simulink model "underactuated_model"  (R2023b)
settings: Solver=VariableStepAuto  StartTime=0.0  StopTime=10.0  RelTol=1e-6
values from neighbouring files (symbols this model uses):
  h0 = 0.3    [how_do_limits_affect_convergence.m]    (also in run_underactuated_model.m)
settings Model: Creator=Aaron  LastModifiedBy=Aaron

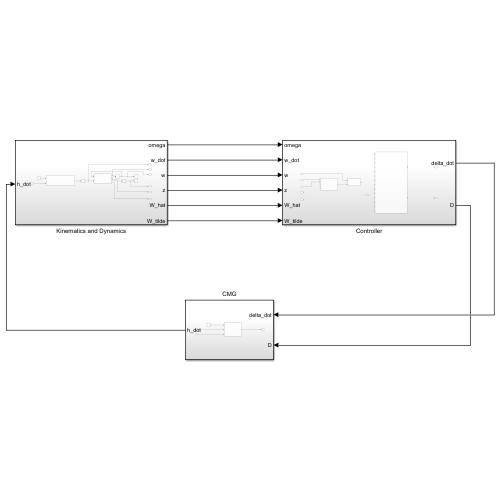
[thumbnail: Simulink's stored preview of the top-level diagram]
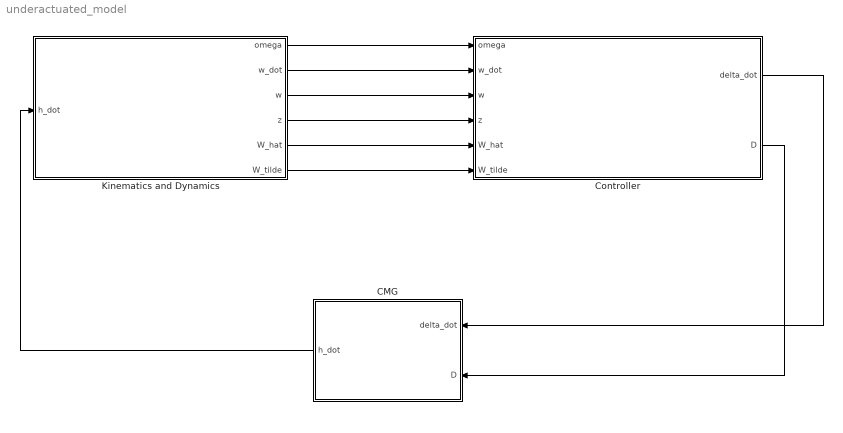
== system underactuated_model ==
  CMG : Subsystem
  Controller : Subsystem
  Kinematics and Dynamics : Subsystem
  wires:
  Kinematics and Dynamics/1(omega) -> Controller/1(omega)
  Kinematics and Dynamics/3(w) -> Controller/3(w)
  Kinematics and Dynamics/4(z) -> Controller/4(z)
  Kinematics and Dynamics/2(w_dot) -> Controller/2(w_dot)
  Kinematics and Dynamics/5(W_hat) -> Controller/5(W_hat)
  Kinematics and Dynamics/6(W_tilde) -> Controller/6(W_tilde)
  Controller/1(delta_dot) -> CMG/1(delta_dot)
  Controller/2(D) -> CMG/2(D)
  CMG/1(h_dot) -> Kinematics and Dynamics/1(h_dot)

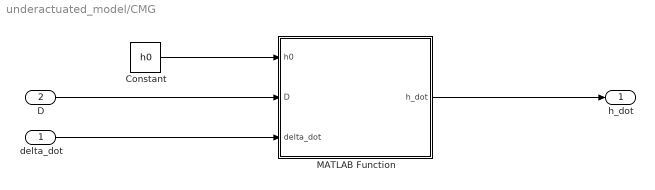
== system underactuated_model/CMG ==
  delta_dot : Inport
  D : Inport  Port=2
  Constant : Constant  Value=h0
  MATLAB Function : MATLAB Function  TreatAsAtomicUnit=on
  h_dot : Outport
  wires:
  delta_dot/1 -> MATLAB Function/3(delta_dot)
  D/1 -> MATLAB Function/2(D)
  MATLAB Function/1(h_dot) -> h_dot/1
  Constant/1 -> MATLAB Function/1(h0)

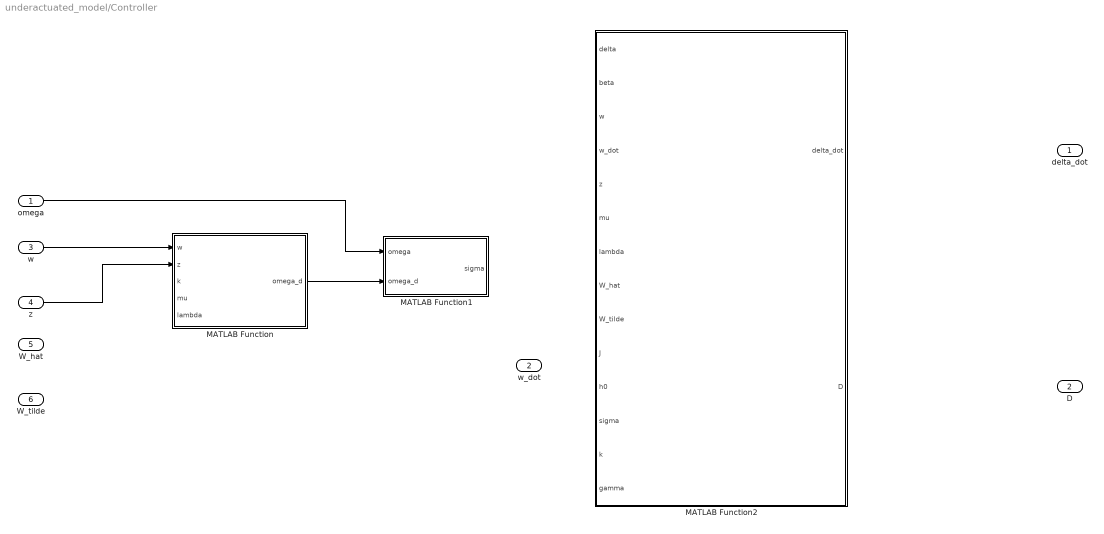
== system underactuated_model/Controller ==
  omega : Inport
  w_dot : Inport  Port=2
  w : Inport  Port=3
  z : Inport  Port=4
  W_hat : Inport  Port=5
  W_tilde : Inport  Port=6
  MATLAB Function : MATLAB Function  TreatAsAtomicUnit=on
  MATLAB Function1 : MATLAB Function  TreatAsAtomicUnit=on
  MATLAB Function2 : MATLAB Function  TreatAsAtomicUnit=on
  delta_dot : Outport
  D : Outport  Port=2
  wires:
  w/1 -> MATLAB Function/1(w)
  z/1 -> MATLAB Function/2(z)
  MATLAB Function/1(omega_d) -> MATLAB Function1/2(omega_d)
  omega/1 -> MATLAB Function1/1(omega)

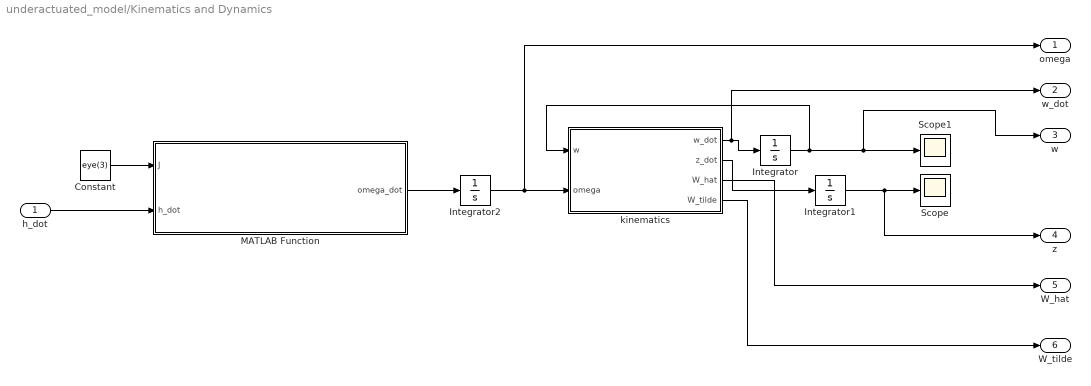
== system underactuated_model/Kinematics and Dynamics ==
  h_dot : Inport
  Constant : Constant  Value=eye(3)
  Integrator : Integrator  InitialCondition=[0;0]
  Integrator1 : Integrator
  Integrator2 : Integrator  InitialCondition=[0;0;0]
  MATLAB Function : MATLAB Function  TreatAsAtomicUnit=on
  Scope : Scope
  Scope1 : Scope
  kinematics : MATLAB Function  TreatAsAtomicUnit=on
  omega : Outport
  w_dot : Outport  Port=2
  w : Outport  Port=3
  z : Outport  Port=4
  W_hat : Outport  Port=5
  W_tilde : Outport  Port=6
  wires:
  Integrator2/1 -> omega/1, kinematics/2(omega)
  MATLAB Function/1(omega_dot) -> Integrator2/1
  Integrator1/1 -> z/1, Scope/1
  kinematics/2(z_dot) -> Integrator1/1
  Constant/1 -> MATLAB Function/1(J)
  h_dot/1 -> MATLAB Function/2(h_dot)
  kinematics/1(w_dot) -> w_dot/1, Integrator/1
  Integrator/1 -> kinematics/1(w), w/1, Scope1/1
  kinematics/3(W_hat) -> W_hat/1
  kinematics/4(W_tilde) -> W_tilde/1

== matlab function underactuated_model/Kinematics and Dynamics/MATLAB Function ==
  data: J input; h_dot input; omega_dot output
function omega_dot  = equations_of_motion(J, h_dot)
    % Equation (15)
    omega_dot = -J \ h_dot;
end

== matlab function underactuated_model/Kinematics and Dynamics/kinematics ==
  data: w input; w_dot output; omega input; z_dot output; W_hat output; W_tilde output
function [w_dot, z_dot, W_hat, W_tilde] = kinematics(w, omega)
    w1 = w(1);
    w2 = w(2);
    W =  [(1 + w1^2 - w2^2)/2, w1*w2, w2;
     w1*w2, (1 - w1^2 + w2^2)/2, -w1;
     -w2, w1, 1];

    res = W * omega;

    w_dot = [res(1); res(2)];
    z_dot = res(3);

    W_hat = W(1:2, :);
    W_tilde = W(3, :);

end

== matlab function underactuated_model/Controller/MATLAB Function ==
  data: w input; omega_d output; z input; k input; mu input; lambda input
function omega_d = desired_ang_vel(w, z, k, mu, lambda)

omega_d = (-k/sqrt(1+norm(w)^2)) * [w(1); w(2)] + ...
((mu * (z+lambda*omega(3)))/(w(1)^2 + w(2)^2)) * [w(2); -w(1)];

end

== matlab function underactuated_model/Controller/MATLAB Function1 ==
  data: omega input; sigma output; omega_d input
function sigma = fcn(omega, omega_d)

sigma = [omega(1); omega(2)] - omega_d;

== matlab function underactuated_model/Controller/MATLAB Function2 ==
  data: delta input; delta_dot output; beta input; w input; w_dot input; z input; mu input; lambda input; W_hat input; W_tilde input; J input; h0 input; sigma input; k input; gamma input; D output
function [delta_dot, D] = steering_law(delta, beta, w, w_dot, z, mu, lambda, W_hat, W_tilde, J, h0, sigma, k, gamma)
    D = calc_D(delta, beta);
    D_hat = D(1:2, 1:2);
    D_tilde = D(3, 1:2);

    f1 = calc_f1(w);
    f2 = calc_f2(w, mu, lambda);
    g1 = calc_g1(w, w_dot, z, omega, W_tilde, W_hat);
    g2 = calc_g2(w, z);

    D_fancy = inv(J(1:2, 1:2)) * D_hat + J(3, 3) * f2 * D_tilde'

    delta_dot = (1/h0) * inv(D_fancy) * (gamma*sigma + k*f1*[W_hat; W_tilde]*omega + g1 + g2);

end

function D = calc_D(delta, beta)
    D = [-cos(beta)*cos(delta(1)) cos(beta)*cos(delta(3));
            sin(beta)*cos(delta(1)) sin(beta) * cos(delta(3));
            sin(delta(1)) -sin(delta(3))];
end

function f1 = calc_f1(w)
    f1 = (1/sqrt(1+norm(w)^2)^3) * [1+w(2)^2, -w(1)*w(2); -w(1)*w(2), 1+w(1)^2];
end

function f2 = calc_f2(w, mu, lambda)
    f2 = -(mu * lambda)/(w(1)^2 + w(2)^2) * [w(2); -w(1)];
end

function g1 = calc_g1(w, w_dot, z, omega, W_tilde, W_hat)
    w_tilde = [w(2); -w(1)];
    w_dot_tilde = [w_dot(2); -w_dot(1)];

    first_term = -(mu * W_tilde * omega)/(norm(w)^2) * w_tilde;

    second_term = -(mu*(z+lambda*omega(3)))/(norm(w)^2) * w_dot_tilde;

    third_term = (2*mu*(z+lambda*omega(3) * w' * W_hat * omega))/(norm(w)^4) * w_tilde;

    g1 = first_term + second_term + third_term;
end

function g2 = calc_g2(w, z)
    w_tilde = [w(2); -w(1)];

    g2 = sqrt(1+norm(w)^2) * w - z*w_tilde;
end

== matlab function underactuated_model/CMG/MATLAB Function ==
  data: h0 input; h_dot output; D input; delta_dot input
function h_dot = calc_h_dot(h0, D, delta_dot)
    h_dot = h0 * D * delta_dot;

end
